simulink model "custom_uav_blocks"  (R2023b)
settings: Solver=VariableStepAuto  StartTime=0.0  StopTime=10  RelTol=1e-3
libraries: simulink x6, uavutilslib x1
settings Model: Creator=rakshan  LastModifiedBy=rakshan

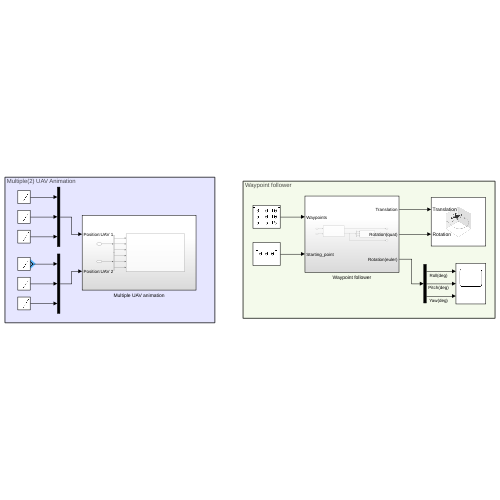
[thumbnail: Simulink's stored preview of the top-level diagram]
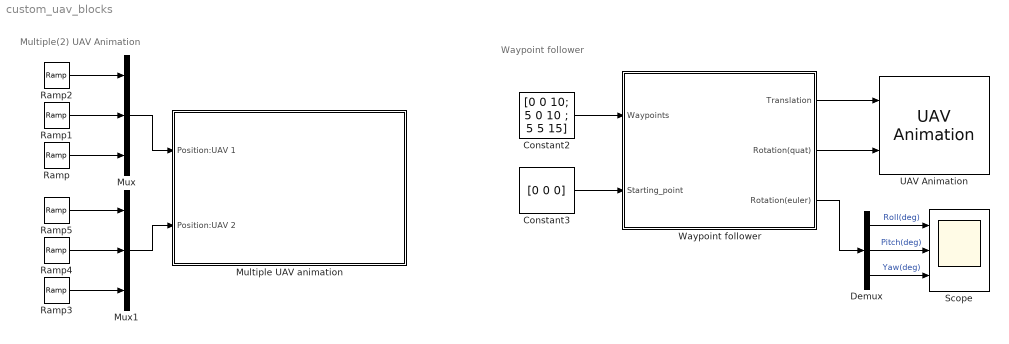
== system custom_uav_blocks ==
  note: Waypoint follower
  note: Multiple(2) UAV Animation
  Constant2 : Constant  Value=[0 0 10; 5 0 10 ; 5 5 15]
  Constant3 : Constant  Value=[0 0 0]  VectorParams1D=off
  Demux : Demux  Outputs=3
  Multiple UAV animation : Subsystem
  Mux : Mux  Inputs=3
  Mux1 : Mux  Inputs=3
  Ramp{,1..4} (5 alike) : simulink/Sources/Ramp  slope=1  start=0  InitialOutput=0
  Ramp5 : simulink/Sources/Ramp  slope=-1  start=0  InitialOutput=0
  Scope : Scope  NumInputPorts=3
  UAV Animation : uavutilslib/UAV Animation  UAVType=Multirotor  UAVSize=4  InertialZDirection=Up  SampleTime=-1
  Waypoint follower : Subsystem
  wires:
  Constant2/1 -> Waypoint follower/1(Waypoints)
  Constant3/1 -> Waypoint follower/2(Starting_point)
  Waypoint follower/1(Translation) -> UAV Animation/1
  Waypoint follower/2(Rotation(quat)) -> UAV Animation/2
  Demux/1 -> Scope/1  "Roll(deg)"
  Demux/2 -> Scope/2  "Pitch(deg)"
  Demux/3 -> Scope/3  "Yaw(deg)"
  Waypoint follower/3(Rotation(euler)) -> Demux/1
  Ramp1/1 -> Mux/2
  Ramp2/1 -> Mux/1
  Ramp/1 -> Mux/3
  Mux/1 -> Multiple UAV animation/1(Position:UAV 1)
  Ramp3/1 -> Mux1/3
  Ramp5/1 -> Mux1/1
  Ramp4/1 -> Mux1/2
  Mux1/1 -> Multiple UAV animation/2(Position:UAV 2)

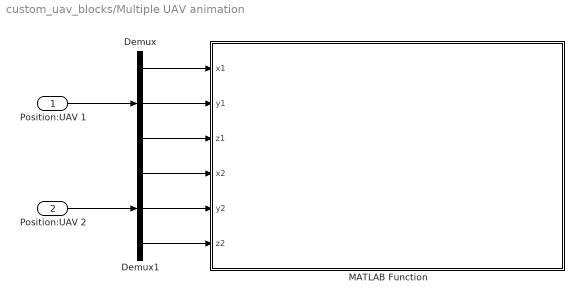
== system custom_uav_blocks/Multiple UAV animation ==
  Position:UAV 1 : Inport
  Position:UAV 2 : Inport  Port=2
  Demux : Demux  Outputs=3
  Demux1 : Demux  Outputs=3
  MATLAB Function : MATLAB Function  TreatAsAtomicUnit=on
  wires:
  Demux/1 -> MATLAB Function/1(x1)
  Demux/2 -> MATLAB Function/2(y1)
  Demux/3 -> MATLAB Function/3(z1)
  Demux1/1 -> MATLAB Function/4(x2)
  Demux1/2 -> MATLAB Function/5(y2)
  Demux1/3 -> MATLAB Function/6(z2)
  Position:UAV 2/1 -> Demux1/1
  Position:UAV 1/1 -> Demux/1

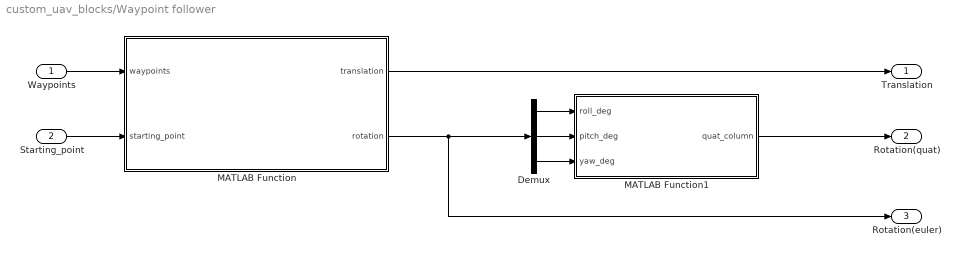
== system custom_uav_blocks/Waypoint follower ==
  Waypoints : Inport
  Starting_point : Inport  Port=2
  Demux : Demux  Outputs=3
  MATLAB Function : MATLAB Function  TreatAsAtomicUnit=on
  MATLAB Function1 : MATLAB Function  TreatAsAtomicUnit=on
  Translation : Outport
  Rotation(quat) : Outport  Port=2
  Rotation(euler) : Outport  Port=3
  wires:
  Demux/1 -> MATLAB Function1/1(roll_deg)
  Demux/3 -> MATLAB Function1/3(yaw_deg)
  Demux/2 -> MATLAB Function1/2(pitch_deg)
  MATLAB Function1/1(quat_column) -> Rotation(quat)/1
  MATLAB Function/2(rotation) -> Rotation(euler)/1, Demux/1
  Waypoints/1 -> MATLAB Function/1(waypoints)
  Starting_point/1 -> MATLAB Function/2(starting_point)
  MATLAB Function/1(translation) -> Translation/1

== matlab function custom_uav_blocks/Waypoint follower/MATLAB Function ==
  data: waypoints input; translation output; rotation output; starting_point input
function [translation, rotation] = interpolateWaypointsSimulink(waypoints,starting_point)
    persistent current_waypoint;
    persistent current_index;
    time_step = 0.4;
   
    waypoints = [starting_point;waypoints]
    % Initialize persistent variables on first call
    if isempty(current_waypoint)
        current_waypoint = waypoints(1,:);
        current_index = 1;
    end
    
    % Initialize outputs
    translation = zeros(1, 3);
    rotation = zeros(1, 3); % Euler angles: [yaw, pitch, roll]
    
    % Check if reached last waypoint
    if current_index == size(waypoints, 1)
        translation = waypoints(end, :);
        rotation = [0 0 0]; % No rotation (identity)
    else
        % Interpolate translation
        translation = current_waypoint;
        next_waypoint = waypoints(current_index + 1, :);
        current_waypoint = current_waypoint + (next_waypoint - current_waypoint) * time_step;
        
        % Calculate direction vector
        direction_vector = next_waypoint - current_waypoint;
        direction_vector = direction_vector / norm(direction_vector); % Normalize
        
        % Calculate rotation angles (Euler angles)
        yaw = atan2(direction_vector(2), direction_vector(1));
        pitch = asin(direction_vector(3));
        roll = 0; % Assuming no roll motion
        
        % Update rotation
        rotation = [yaw pitch roll];
        
        % Check if reached next waypoint
        if norm(current_waypoint - next_waypoint) < 0.01
            current_index = current_index + 1;
        end
    end
end

== matlab function custom_uav_blocks/Waypoint follower/MATLAB Function1 ==
  data: roll_deg input; quat_column output; pitch_deg input; yaw_deg input
function quat_column = eulerToQuat(roll_deg, pitch_deg, yaw_deg)
    % Convert Euler angles to radians
    roll_rad = deg2rad(roll_deg);
    pitch_rad = deg2rad(pitch_deg);
    yaw_rad = deg2rad(yaw_deg);

    % Calculate half angles
    roll_half = roll_rad / 2;
    pitch_half = pitch_rad / 2;
    yaw_half = yaw_rad / 2;

    % Calculate trigonometric functions
    roll_sin = sin(roll_half);
    roll_cos = cos(roll_half);
    pitch_sin = sin(pitch_half);
    pitch_cos = cos(pitch_half);
    yaw_sin = sin(yaw_half);
    yaw_cos = cos(yaw_half);

    % Calculate quaternion components
    q0 = roll_cos * pitch_cos * yaw_cos + roll_sin * pitch_sin * yaw_sin;
    q1 = roll_sin * pitch_cos * yaw_cos - roll_cos * pitch_sin * yaw_sin;
    q2 = roll_cos * pitch_sin * yaw_cos + roll_sin * pitch_cos * yaw_sin;
    q3 = roll_cos * pitch_cos * yaw_sin - roll_sin * pitch_sin * yaw_cos;

    % Format the quaternion as a column vector
    quat_column = [q0; q1; q2; q3];
end

== matlab function custom_uav_blocks/Multiple UAV animation/MATLAB Function ==
  data: x1 input; y1 input; z1 input; x2 input; y2 input; z2 input
% uav_animation.m
function uav_animation(x1, y1, z1, x2, y2, z2)
    persistent traj_x1 traj_y1 traj_z1 traj_x2 traj_y2 traj_z2;
    
    % Initialize the figure
    figure(1);
    clf;
    hold on;
    axis equal;
    grid on;
    xlabel('X');
    ylabel('Y');
    zlabel('Z');
    legend;
    
    % Define a simple UAV shape (e.g., a cuboid)
    [x, y, z] = create_uav_shape();
    
    % Append current positions to the trajectory arrays
    if isempty(traj_x1)
        traj_x1 = x1;
        traj_y1 = y1;
        traj_z1 = z1;
        traj_x2 = x2;
        traj_y2 = y2;
        traj_z2 = z2;
    else
        traj_x1 = [traj_x1 x1];
        traj_y1 = [traj_y1 y1];
        traj_z1 = [traj_z1 z1];
        traj_x2 = [traj_x2 x2];
        traj_y2 = [traj_y2 y2];
        traj_z2 = [traj_z2 z2];
    end

    % Plot UAV1
    surf(x + x1, y + y1, z + z1, 'FaceColor', 'r', 'EdgeColor', 'none','DisplayName',"UAV 1");
    
    % Plot UAV2
    surf(x + x2, y + y2, z + z2, 'FaceColor', 'b', 'EdgeColor', 'none',"DisplayName","UAV 2");

    % Plot trajectory for UAV1
    plot3(traj_x1, traj_y1, traj_z1, '--r', 'LineWidth', 1, 'DisplayName', 'Trajectory: UAV 1');
    
    % Plot trajectory for UAV2
    plot3(traj_x2, traj_y2, traj_z2, '--b', 'LineWidth', 1, 'DisplayName', 'Trajectory: UAV 2');
    
    view(3); % Set the view to 3D
    drawnow;
end

function [x, y, z] = create_uav_shape()
    % Create a simple cuboid shape for the UAV
    [x, y, z] = ndgrid([-0.5, 0.5], [-0.5, 0.5], [-0.1, 0.1]);
    
    % Convert to surface coordinates
    x = reshape(x, [2, 2, 2]);
    y = reshape(y, [2, 2, 2]);
    z = reshape(z, [2, 2, 2]);

    % Create the faces of the cuboid
    x = [x(:, :, 1); x(:, :, 2)];
    y = [y(:, :, 1); y(:, :, 2)];
    z = [z(:, :, 1); z(:, :, 2)];
end
